simulink model "OccupancyGridSimulation"  (R2023a)
settings: Solver=VariableStepAuto  StartTime=0.0  StopTime=5  RelTol=1e-3
undefined symbols (not defined in the file or in its folder): gray
libraries: sim3dcameralib x2, simulink x1, sim3dlib x1, uavsim3dlib x1
settings Model: Creator=hoyos  LastModifiedBy=NEENA
settings OptimizationCC: ReuseModelBlockBuffer=off
settings ModelReferenceCC: EnableRefExpFcnMdlSchedulingChecks=on
settings SFSimCC: SimTargetLang=C++

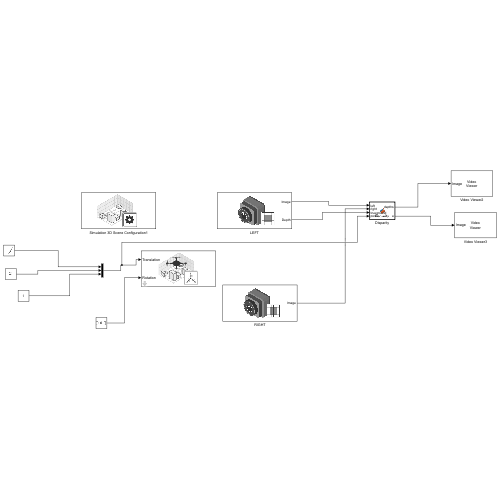
[thumbnail: Simulink's stored preview of the top-level diagram]
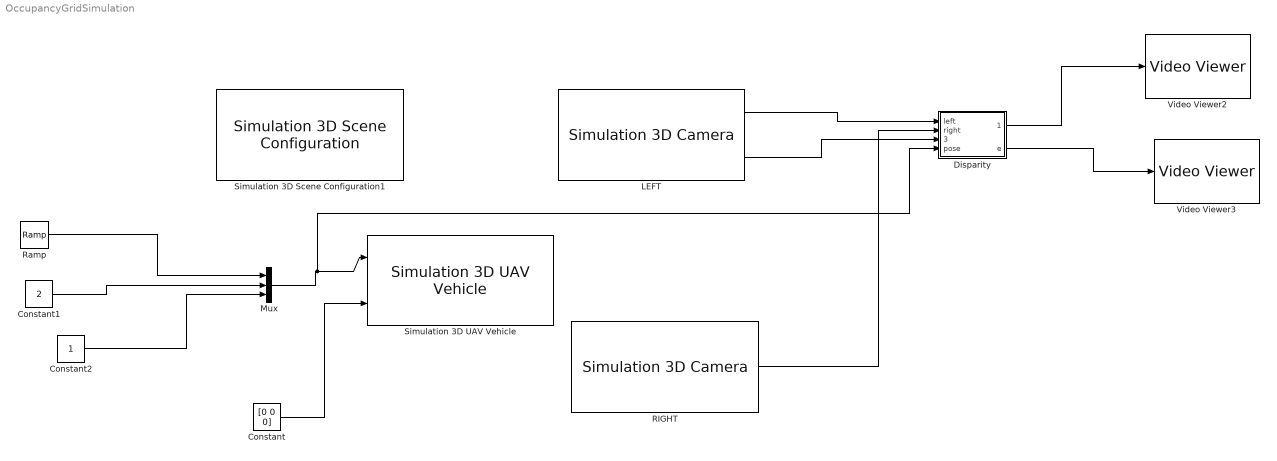
== system OccupancyGridSimulation ==
  Constant : Constant  Value=[0 0 0]
  Constant1 : Constant  Value=2
  Constant2 : Constant
  Disparity : MATLAB Function  TreatAsAtomicUnit=on
  LEFT : sim3dcameralib/Simulation 3D Camera  Priority=1  sensorTag=Sim3dSensor1  sensorId=1  sensorName=Sim3dSensor1  vehTagList={'Quad1';'Scene Origin'}  vehTag=Quad1  mountLoc=Origin  offsetFlag=on  tmountOffset=[0.1, 1/2, 0]  extTmount=off  rmountOffset=[0, 0, 0]  extRmount=off  FocalLength=[1109, 1109]  OpticalCenter=[640, 360]  ImageSize=[720, 1280]  RadialDistortion=[0, 0]  TangentialDistortion=[0, 0]  SensorSkew=0  DepthOutportEnabled=on  SemanticOutportEnabled=off  TransformOutportEnabled=off  SampleTime=-1  mountPoint=[0.1 -0.5 0]  mountOrientation=[0 0 0]  aMode=3  ID=1
  Mux : Mux  Inputs=3
  RIGHT : sim3dcameralib/Simulation 3D Camera  Priority=1  sensorTag=Sim3dSensor2  sensorId=2  sensorName=Sim3dSensor2  vehTagList={'Quad1';'Scene Origin'}  vehTag=Quad1  mountLoc=Origin  offsetFlag=on  tmountOffset=[0.1, -1/2, 0]  extTmount=off  rmountOffset=[0, 0, 0]  extRmount=off  FocalLength=[1109, 1109]  OpticalCenter=[640, 360]  ImageSize=[720, 1280]  RadialDistortion=[0, 0]  TangentialDistortion=[0, 0]  SensorSkew=0  DepthOutportEnabled=off  SemanticOutportEnabled=off  TransformOutportEnabled=off  SampleTime=-1  mountPoint=[0.1 0.5 0]  mountOrientation=[0 0 0]  aMode=3  ID=2
  Ramp : simulink/Sources/Ramp  slope=5  start=0  InitialOutput=0
  Simulation 3D Scene Configuration1 : sim3dlib/Simulation 3D Scene Configuration  Priority=0  ProjectFormat=Default Scenes  SceneDesc=US city block  ProjectName=C:\Program Files\MATLAB\R2023a\toolbox\shared\sim3d_projects\automotive_project\UE4\WindowsNoEditor\VehicleSimulation.exe  ScenePath=/Game/Maps/USCityBlock  EnableOpenDRIVE=off  vehTagList={'Quad1';'Scene Origin'}  vehTag=Quad1  OpVisEn=off  Ts=1/10  EnableWindow=on  EnableRemoteAccess=off  EnableWeather=off  SunAltitude=40.0  SunAzimuth=90  clouds=10  wind=1  fog=0  rain=0  EnableGeospatial=off  OriginHeight=200  OriginLatitude=40.744652  OriginLongitude=-73.988864  MapStyle=Aerial  AdditionalAssetIDs=[]  UseAdvancedSunSky=off  SolarTime=11  TimeZone=-5  Day=21  Month=9  Year=2022  UseDaylightSavingTime=on  DSTStartDay=10  DSTStartMonth=3  DSTEndDay=3  DSTEndMonth=11  DSTSwitchHour=2  sensorTag=MainCamera2  sensorId=2  sensorName=MainCamera2  mountLoc=Origin  offsetFlag=off  tmountOffset=[0, 0, 0]  rmountOffset=[0, 0, 0]  HorizontalResolution=1280  VerticalResolution=720  HorizontalFOV=60  mountPoint=[0 0 0]  mountOrientation=[0 0 0]  aMode=4  ID=2  GeoTrigger=Inactive
  Simulation 3D UAV Vehicle : uavsim3dlib/Simulation 3D UAV Vehicle  Priority=-1  Mesh=Quadrotor  MeshPath=/MathWorksUAVContent/UAVs/HexaRotorUAV/HexaRotor.HexaRotor  Color=Orange  ActorName=Quad1  UseGlobalFrame=off  InitialTranslation=[0 2 1]  InitialRotation=[0 0 0]  InitialTranslationGlobal=[0 0 0]  InitialGeoOrigin=[0 0 0]  InitialRotationGlobal=[0 0 0]  SampleTime=-1  ActorType=SimulinkVehicle  ID=C  aMode=4  ActorTag=Quad1
  Video Viewer2 : VideoViewer  colormapValue=gray(256)  FigPos=[-60.6 693.2 673.6 588]
  Video Viewer3 : VideoViewer  FigPos=[316.2 947.6 766.4 756]
  wires:
  Constant1/1 -> Mux/2
  Constant2/1 -> Mux/3
  Mux/1 -> Disparity/4(pose), Simulation 3D UAV Vehicle/1
  Constant/1 -> Simulation 3D UAV Vehicle/2
  Ramp/1 -> Mux/1
  LEFT/1 -> Disparity/1(left)
  RIGHT/1 -> Disparity/2(right)
  Disparity/1(depths) -> Video Viewer2/1
  LEFT/2 -> Disparity/3(trueground)
  Disparity/2(e) -> Video Viewer3/1

== matlab function OccupancyGridSimulation/Disparity ==
  data: left input; depths output; right input; trueground input; e output; pose input
function [depths,e] = Disparity(left,right,trueground,pose)

depthstereo = uint8(ones(720,1280,3));

error = uint8(ones(720,1280,3));
coder.extrinsic('DisparityMatlab2');

 
[depthstereo error]=DisparityMatlab2(left,right,trueground,pose);




depths = depthstereo;
e=error;
